simulink model "Model_GBXCluctchOpt_V5"  (R2024b)
settings: Solver=VariableStepAuto  StartTime=0.0  StopTime=552  RelTol=1e-5
undefined symbols (not defined in the file): Bdy_facCoG_C, Bdy_facTireFric_C, Bdy_lenRadiusWheel_C, Bdy_lenWheelBase_C, Bdy_lenZCoG_C, Bdy_mEquivalentJ_C, Bdy_mVeh_C, Bdy_vsqr2frc_C, Drv_kmh2gradtqDriver_C, Drv_kmh2tqDriver_C, Edr_pwr_LossMap_AXIS, Edr_pwrInverterLosses_MAP, Edr_pwrMachineLosses_MAP, Edr_rpm_InvLossMap_AXIS, Edr_rpm_MachLossMap_AXIS, Edr_rpm_MaxMinTq_AXIS, Edr_rpmMax_C, Edr_tq_MachLossMap_AXIS, Edr_tqEffMax_CUR, Env_facSlope_WLTC_CUR, Env_facSlopeBAB185_CUR, Env_facSlopeCrossCountry_CUR, Env_kmhDesBAB185_CUR, Env_kmhDesCrossCountry_CUR, Env_vVehDes_NEDC_kmh, Env_vVehDes_WLTC_kmh, Env_vVehTime_NEDC_s, Env_vVehTime_WLTC_s, Gbx_facGbxRatioRe_C, Ice_derfacLoadDecrease_MAP, Ice_derfacLoadIncrease_MAP, Ice_etaLam_CUR, Ice_facEtaCocMax_MAP, Ice_facFuelEnRich_MAP, Ice_KUMSRL_C, Ice_Lambda_AXIS, Ice_relLoad2relTqOptIgnLamOne_MAP, Ice_relLoad_AXIS, Ice_relLoad_LoadDyn_AXIS, Ice_relLoad_Max_CUR, Ice_relTq_AXIS, Ice_relTqInr2TqInr_C, Ice_relTqOptIgnLamOne2relLoad_MAP, Ice_rpm_AXIS, Ice_rpm_LoadDyn_AXIS, Ice_rpm_relLoadMax_AXIS, Ice_tqLossesIce_MAP, Pnt_capBat_C, Pnt_facSocBatOcv_AXIS, Pnt_facSocInit_C, Pnt_iBatChrgMax_C, Pnt_iBatDisChrgMax_C, Pnt_resBatInner_C, Pnt_uBatMax_C, Pnt_uBatMin_C, Pnt_uBatOcv_CUR, Vco_flgEdrExists_CFG, Vco_flgIceCluAlwClosed_CFG, Vco_flgIceExists_CFG
libraries: simulink x7, simulink_extras x6
(part 2 of 3)

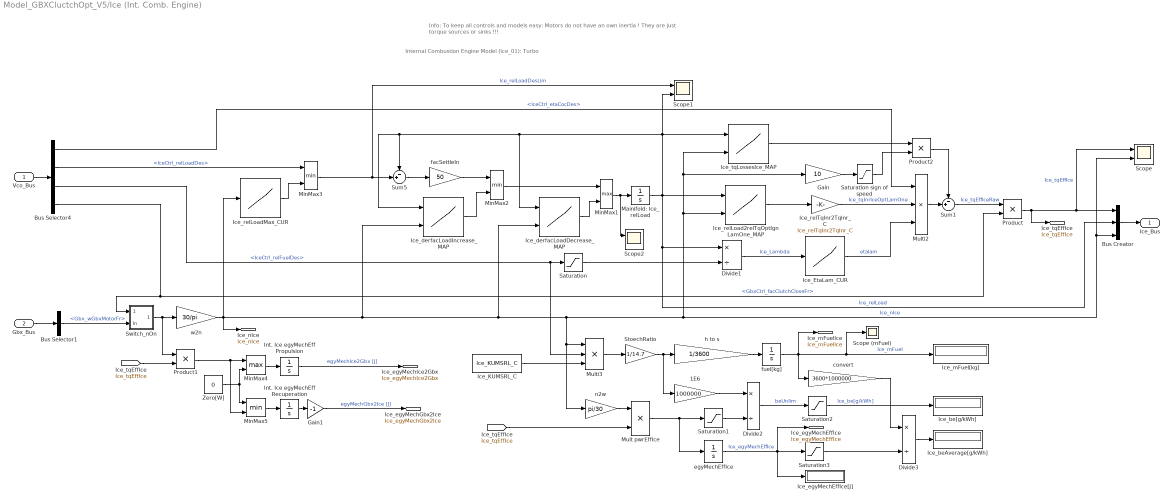
== system Model_GBXCluctchOpt_V5/Ice (Int. Comb. Engine) ==
  note: Internal Combustion Engine Model (Ice_01): Turbo
  note: Info: To keep all controls and models easy: Motors do not have an own inertia !
      | They are just torque sources or sinks !!!
  Vco_Bus : Inport
  Gbx_Bus : Inport  Port=2
  " h to s" : Gain  Gain=1/3600
  1E6 : Gain  Gain=1000000
  Bus Creator : BusCreator  Inputs=3
  Bus Selector1 : BusSelector  OutputSignals=Gbx_wGbxMotorFr
  Bus Selector4 : BusSelector  OutputSignals=IceCtrl_etaCocDes,IceCtrl_relLoadDes,IceCtrl_relFuelDes,GbxCtrl_facClutchCloseFr
  Divide1 : Product  Inputs=*/
  Divide2 : Product  Inputs=*/
  Divide3 : Product  Inputs=*/
  Gain : Gain  Gain=10
  Gain1 : Gain  Gain=-1
  Ice_EtaLam_CUR : Lookup_n-D  NumberOfTableDimensions=1  BreakpointsForDimension1=Ice_Lambda_AXIS  Table=Ice_etaLam_CUR  ExtrapMethod=Clip  InternalRulePriority=Speed  RndMeth=Simplest
  Ice_KUMSRL_C : Constant  Value=Ice_KUMSRL_C
  Ice_beAverage[g/kWh] : Display
  Ice_be[g/kWh] : Display
  Ice_derfacLoadDecrease_MAP : Lookup_n-D  BreakpointsForDimension1=Ice_relLoad_LoadDyn_AXIS  BreakpointsForDimension2=Ice_rpm_LoadDyn_AXIS  Table=Ice_derfacLoadDecrease_MAP  ExtrapMethod=Clip  UseLastTableValue=on  InternalRulePriority=Speed  RndMeth=Simplest
      settings: InputPortMap=u0,u1
  Ice_derfacLoadIncrease_MAP : Lookup_n-D  BreakpointsForDimension1=Ice_relLoad_LoadDyn_AXIS  BreakpointsForDimension2=Ice_rpm_LoadDyn_AXIS  Table=Ice_derfacLoadIncrease_MAP  ExtrapMethod=Clip  UseLastTableValue=on  InternalRulePriority=Speed  RndMeth=Simplest
      settings: InputPortMap=u0,u1
  Ice_egyMechEffIce[J] : Display
  Ice_mFuel[kg] : Display
  Ice_relLoad2relTqOptIgnLamOne_MAP : Lookup_n-D  BreakpointsForDimension1=Ice_relLoad_AXIS  BreakpointsForDimension2=Ice_rpm_AXIS  Table=Ice_relLoad2relTqOptIgnLamOne_MAP  ExtrapMethod=Clip  InternalRulePriority=Speed  RndMeth=Simplest
      settings: InputPortMap=u0,u1
  Ice_relLoadMax_CUR : Lookup_n-D  NumberOfTableDimensions=1  BreakpointsForDimension1=Ice_rpm_relLoadMax_AXIS  Table=Ice_relLoad_Max_CUR  ExtrapMethod=Clip  InternalRulePriority=Speed  RndMeth=Simplest
  Ice_relTqInr2TqInr_C : Gain  Gain=Ice_relTqInr2TqInr_C
  Ice_tqLossesIce_MAP : Lookup_n-D  BreakpointsForDimension1=Ice_relLoad_AXIS  BreakpointsForDimension2=Ice_rpm_AXIS  Table=Ice_tqLossesIce_MAP  ExtrapMethod=Clip  InternalRulePriority=Speed  RndMeth=Simplest
      settings: InputPortMap=u0,u1
  Int. Ice egyMechEff Propulsion : Integrator
  Int. Ice egyMechEff Recuperation : Integrator
  Mainifold: Ice_relLoad : Integrator  InitialCondition=80  LimitOutput=on  LowerSaturationLimit=0
  MinMax1 : MinMax  Function=max  Inputs=2
  MinMax2 : MinMax  Inputs=2
  MinMax3 : MinMax  Inputs=2
  MinMax4 : MinMax  Function=max  Inputs=2  ZeroCross=off
  MinMax5 : MinMax  Inputs=2  ZeroCross=off
  Mult pwrEffIce : Product  Inputs=**
  Multi2 : Product  Inputs=***
  Multi3 : Product  Inputs=***
  Product : Product
  Product1 : Product
  Product2 : Product
  Saturation : Saturate  UpperLimit=1000  LowerLimit=0.0001
  Saturation sign of speed : Saturate  UpperLimit=1  LowerLimit=-1
  Saturation1 : Saturate  UpperLimit=inf  LowerLimit=0.1
  Saturation2 : Saturate  UpperLimit=1000  LowerLimit=0
  Saturation3 : Saturate  UpperLimit=inf  LowerLimit=0.1
  Scope : Scope  NumInputPorts=2
  "Scope (mFuel) " : Scope
  Scope1 : Scope  NumInputPorts=2
  Scope2 : Scope  NumInputPorts=2
  StoechRatio : Gain  Gain=1/14.7
  Sum1 : Sum  Inputs=-+|
  Sum5 : Sum  Inputs=-+|
  Switch_nOn : Subsystem
  "Zero[W] " : Constant  Value=0
  convert : Gain  Gain=3600*1000000
  egyMechEffIce : Integrator
  facSettleIn : Gain  Gain=50
  fuel[kg] : Integrator
  n2w : Gain  Gain=pi/30
  "w2n  " : Gain  Gain=30/pi
  Ice_Bus : Outport  VectorParamsAs1DForOutWhenUnconnected=off
  tag scope: Ice_egyMechEffIce=global, Ice_egyMechGbx2Ice=global, Ice_egyMechIce2Gbx=global, Ice_mFuelIce=global, Ice_nIce=global, Ice_tqEffIce=global
  wires:
  Bus Creator/1 -> Ice_Bus/1
  Vco_Bus/1 -> Bus Selector4/1
  Product/1 -> [Ice_tqEffIce], Bus Creator/1, Scope/1  "Ice_tqEffIce"
  Gbx_Bus/1 -> Bus Selector1/1
  "w2n  "/1 -> [Ice_nIce], Ice_relLoadMax_CUR/1, Ice_derfacLoadDecrease_MAP/2, n2w/1, Multi3/1, Gain/1, Ice_tqLossesIce_MAP/2, Ice_relLoad2relTqOptIgnLamOne_MAP/2, Scope/2, Bus Creator/3, Ice_derfacLoadIncrease_MAP/2  "Ice_nIce"
  Bus Selector1/1 -> Switch_nOn/2(In)  "<Gbx_wGbxMotorFr>"
  Mainifold: Ice_relLoad/1 -> Bus Creator/2, Divide1/1, Ice_relLoad2relTqOptIgnLamOne_MAP/1, Scope1/2, Ice_tqLossesIce_MAP/1, Ice_derfacLoadDecrease_MAP/1, Ice_derfacLoadIncrease_MAP/1, Sum5/1  "Ice_relLoad"
  Ice_relLoadMax_CUR/1 -> MinMax3/2
  Bus Selector4/2 -> MinMax3/1  "<IceCtrl_relLoadDes>"
  Bus Selector4/1 -> Multi2/1  "<IceCtrl_etaCocDes>"
  Bus Selector4/3 -> Multi3/2, Saturation/1  "<IceCtrl_relFuelDes>"
  Ice_derfacLoadIncrease_MAP/1 -> MinMax2/2
  Ice_derfacLoadDecrease_MAP/1 -> MinMax1/2
  MinMax2/1 -> MinMax1/1
  MinMax1/1 -> Scope2/1, Mainifold: Ice_relLoad/1
  Sum5/1 -> facSettleIn/1
  facSettleIn/1 -> MinMax2/1
  MinMax3/1 -> Scope1/1, Sum5/2  "Ice_relLoadDesLim"
  Saturation/1 -> Divide1/2
  Divide1/1 -> Ice_EtaLam_CUR/1  "Ice_Lambda"
  Ice_relLoad2relTqOptIgnLamOne_MAP/1 -> Ice_relTqInr2TqInr_C/1
  Ice_relTqInr2TqInr_C/1 -> Multi2/2  "Ice_tqInrIceOptLamOne"
  Ice_EtaLam_CUR/1 -> Multi2/3  "etalam"
  Multi2/1 -> Sum1/2
  Ice_tqLossesIce_MAP/1 -> Product2/1
  Sum1/1 -> Product/1  "Ice_tqEffIceRaw"
  Bus Selector4/4 -> Switch_nOn/1(flag), Product/2  "<GbxCtrl_facClutchCloseFr>"
  Int. Ice egyMechEff Recuperation/1 -> Gain1/1
  MinMax5/1 -> Int. Ice egyMechEff Recuperation/1
  "Zero[W] "/1 -> MinMax5/1, MinMax4/2
  Product1/1 -> MinMax4/1, MinMax5/2
  MinMax4/1 -> Int. Ice egyMechEff Propulsion/1
  Gain1/1 -> [Ice_egyMechGbx2Ice]  "egyMechGbx2Ice [J]"
  Int. Ice egyMechEff Propulsion/1 -> [Ice_egyMechIce2Gbx]  "egyMechIce2Gbx [J]"
  [Ice_tqEffIce] -> Product1/2
  Switch_nOn/1(Out) -> Product1/1, "w2n  "/1
  Product2/1 -> Sum1/1
  Saturation sign of speed/1 -> Product2/2
  Gain/1 -> Saturation sign of speed/1
  Ice_KUMSRL_C/1 -> Multi3/3
  Multi3/1 -> StoechRatio/1
  StoechRatio/1 -> 1E6/1, " h to s"/1
  " h to s"/1 -> fuel[kg]/1
  fuel[kg]/1 -> convert/1, [Ice_mFuelIce], "Scope (mFuel) "/1, Ice_mFuel[kg]/1  "Ice_mFuel"
  [Ice_tqEffIce] -> Mult pwrEffIce/2
  n2w/1 -> Mult pwrEffIce/1
  Mult pwrEffIce/1 -> egyMechEffIce/1, Saturation1/1
  Saturation1/1 -> Divide2/2
  1E6/1 -> Divide2/1
  Divide2/1 -> Saturation2/1  "beUnlim"
  Saturation2/1 -> Ice_be[g/kWh]/1  "Ice_be[g/kWh]"
  egyMechEffIce/1 -> [Ice_egyMechEffIce], Ice_egyMechEffIce[J]/1, Saturation3/1  "Ice_egyMechEffIce"
  Saturation3/1 -> Divide3/2
  convert/1 -> Divide3/1
  Divide3/1 -> Ice_beAverage[g/kWh]/1

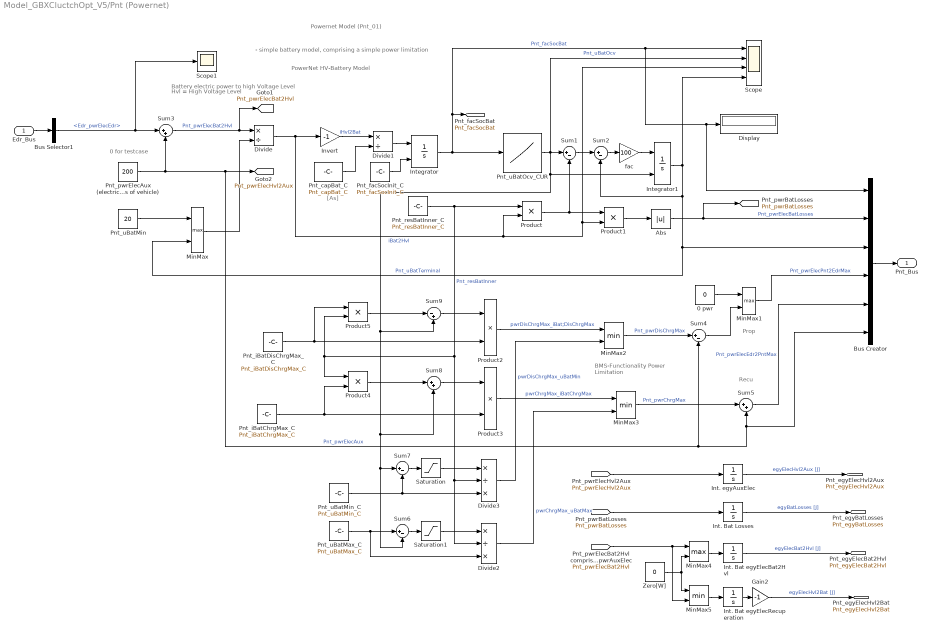
== system Model_GBXCluctchOpt_V5/Pnt (Powernet) ==
  note: Prop
  note: 0 for testcase
  note: [As]
  note: Powernet Model (Pnt_01)
  note: PowerNet HV-Battery Model
  note: Battery electric power to high Voltage Level
  note: Recu
  note: - simple battery model, comprising a simple power limitation
  note: BMS-Functionality
      | Power Limitation
  note: Hvl = High Voltage Level
  Edr_Bus : Inport
  0 pwr : Constant  Value=0
  Abs : Abs  SaturateOnIntegerOverflow=off
  Bus Creator : BusCreator  Inputs=6
  Bus Selector1 : BusSelector  OutputSignals=Edr_pwrElecEdr
  Display : Display
  Divide : Product  Inputs=*/
  Divide1 : Product  Inputs=*/
  Divide2 : Product  Inputs=*/*
  Divide3 : Product  Inputs=*/*
  Gain2 : Gain  Gain=-1
  Int. Bat Losses : Integrator
  Int. Bat egyElecBat2Hvl : Integrator
  Int. Bat egyElecRecuperation : Integrator
  Int. egyAuxElec : Integrator
  Integrator : Integrator  InitialConditionSource=external  InitialCondition=0.8  LimitOutput=on  UpperSaturationLimit=1  LowerSaturationLimit=0
  Integrator1 : Integrator  InitialConditionSource=external  InitialCondition=0.8
  Invert : Gain  Gain=-1
  MinMax : MinMax  Function=max  Inputs=2
  MinMax1 : MinMax  Function=max  Inputs=2
  MinMax2 : MinMax  Inputs=2
  MinMax3 : MinMax  Inputs=2
  MinMax4 : MinMax  Function=max  Inputs=2  ZeroCross=off
  MinMax5 : MinMax  Inputs=2  ZeroCross=off
  Pnt_capBat_C : Constant  Value=Pnt_capBat_C
  Pnt_facSocInit_C : Constant  Value=Pnt_facSocInit_C
  Pnt_iBatChrgMax_C : Constant  Value=Pnt_iBatChrgMax_C
  Pnt_iBatDisChrgMax_C : Constant  Value=Pnt_iBatDisChrgMax_C
  Pnt_pwrElecAux (electric auxilliaries of vehicle) : Constant  Value=200
  Pnt_resBatInner_C : Constant  Value=Pnt_resBatInner_C
  Pnt_uBatMax_C : Constant  Value=Pnt_uBatMax_C
  Pnt_uBatMin : Constant  Value=20
  Pnt_uBatMin_C : Constant  Value=Pnt_uBatMin_C
  Pnt_uBatOcv_CUR : Lookup  InputValues=Pnt_facSocBatOcv_AXIS  Table=Pnt_uBatOcv_CUR  LookUpMeth=Interpolation-Use End Values  SaturateOnIntegerOverflow=off
  Product : Product  RndMeth=Zero
  Product1 : Product  RndMeth=Zero
  Product{2..5} (4 alike) : Product
  Saturation : Saturate  UpperLimit=1000  LowerLimit=0
  Saturation1 : Saturate  UpperLimit=1000  LowerLimit=0
  Scope : Scope  NumInputPorts=4
  Scope1 : Scope
  Sum{1..2,4,6..7} (5 alike) : Sum  Inputs=|+-
  Sum3 : Sum  Inputs=|++
  Sum5 : Sum  Inputs=|++
  Sum8 : Sum  Inputs=|++
  Sum9 : Sum  Inputs=|-+
  Zero[W] : Constant  Value=0
  fac : Gain  Gain=100
  Pnt_Bus : Outport  VectorParamsAs1DForOutWhenUnconnected=off
  tag scope: Pnt_egyBatLosses=global, Pnt_egyElecBat2Hvl=global, Pnt_egyElecHvl2Aux=global, Pnt_egyElecHvl2Bat=global, Pnt_facSocBat=global, Pnt_pwrBatLosses=global, Pnt_pwrElecBat2Hvl=global, Pnt_pwrElecHvl2Aux=global
  wires:
  Bus Creator/1 -> Pnt_Bus/1
  Sum5/1 -> Bus Creator/5  "Pnt_pwrElecEdr2PntMax"
  MinMax1/1 -> Bus Creator/4  "Pnt_pwrElecPnt2EdrMax"
  Int. egyAuxElec/1 -> [Pnt_egyElecHvl2Aux]  "egyElecHvl2Aux [J]"
  Int. Bat Losses/1 -> [Pnt_egyBatLosses]  "egyBatLosses [J]"
  [Pnt_pwrElecHvl2Aux] -> Int. egyAuxElec/1
  Pnt_iBatDisChrgMax_C/1 -> Product5/1, Product2/2
  Sum8/1 -> Product3/1
  Zero[W]/1 -> MinMax5/1, MinMax4/2
  [Pnt_pwrBatLosses] -> Int. Bat Losses/1
  0 pwr/1 -> MinMax1/1
  Pnt_iBatChrgMax_C/1 -> Product4/2, Product3/2
  Saturation1/1 -> Divide2/1
  Pnt_pwrElecAux (electric auxilliaries of vehicle)/1 -> Sum5/2, Bus Creator/6, Sum4/2, [Pnt_pwrElecHvl2Aux], Sum3/2  "Pnt_pwrElecAux"
  Divide/1 -> Invert/1, Product/2, Scope/3, Product1/2  "iBat2Hvl"
  Pnt_uBatMax_C/1 -> Divide2/3, Sum6/1
  MinMax5/1 -> Int. Bat egyElecRecuperation/1
  Sum6/1 -> Saturation1/1
  Gain2/1 -> [Pnt_egyElecHvl2Bat]  "egyElecHvl2Bat [J]"
  Sum1/1 -> Sum2/1
  Int. Bat egyElecRecuperation/1 -> Gain2/1
  Int. Bat egyElecBat2Hvl/1 -> [Pnt_egyElecBat2Hvl]  "egyElecBat2Hvl [J]"
  MinMax/1 -> Divide/2
  Sum3/1 -> [Pnt_pwrElecBat2Hvl], Divide/1  "Pnt_pwrElecBat2Hvl"
  Divide3/1 -> MinMax2/2  "pwrDisChrgMax_uBatMin"
  Product5/1 -> Sum9/1
  Divide2/1 -> MinMax3/2  "pwrChrgMax_uBatMax"
  Sum7/1 -> Saturation/1
  Product4/1 -> Sum8/1
  MinMax4/1 -> Int. Bat egyElecBat2Hvl/1
  Sum2/1 -> fac/1
  Integrator1/1 -> MinMax/2, Bus Creator/3, Sum2/2, Scope/4  "Pnt_uBatTerminal"
  MinMax3/1 -> Sum5/1  "Pnt_pwrChrgMax"
  Product3/1 -> MinMax3/1  "pwrChrgMax_iBatChrgMax"
  Abs/1 -> [Pnt_pwrBatLosses], Bus Creator/2  "Pnt_pwrElecBatLosses"
  MinMax2/1 -> Sum4/1  "Pnt_pwrDisChrgMax"
  Pnt_uBatOcv_CUR/1 -> Scope/2, Sum9/2, Sum8/2, Sum6/2, Sum7/1, Integrator1/2, Sum1/1  "Pnt_uBatOcv"
  fac/1 -> Integrator1/1
  Product2/1 -> MinMax2/1  "pwrDisChrgMax_iBat;DisChrgMax"
  Pnt_resBatInner_C/1 -> Divide2/2, Divide3/2, Product4/1, Product5/2, Product/1  "Pnt_resBatInner"
  Sum9/1 -> Product2/1
  Product/1 -> Product1/1, Sum1/2
  [Pnt_pwrElecBat2Hvl] -> MinMax4/1, MinMax5/2
  Invert/1 -> Divide1/1  "iHvl2Bat"
  Bus Selector1/1 -> Sum3/1, Scope1/1  "<Edr_pwrElecEdr>"
  Integrator/1 -> Pnt_uBatOcv_CUR/1, Display/1, Bus Creator/1, Scope/1, [Pnt_facSocBat]  "Pnt_facSocBat"
  Sum4/1 -> MinMax1/2
  Product1/1 -> Abs/1
  Pnt_uBatMin_C/1 -> Sum7/2, Divide3/3
  Divide1/1 -> Integrator/1
  Saturation/1 -> Divide3/1
  Pnt_uBatMin/1 -> MinMax/1
  Pnt_facSocInit_C/1 -> Integrator/2
  Pnt_capBat_C/1 -> Divide1/2
  Edr_Bus/1 -> Bus Selector1/1

== system Model_GBXCluctchOpt_V5/Vco (Vehicle Control) ==
  note: GbxCtrl shall comprise the calculation of the desired torques for the motors, it shall respect the max. torque that can be transferred to the road.
  note: Vehicle Control Model (Vco_Hybrid_01)
      | Variant - for P4 Hybrid with
      | - Rear Axel Central Drive, Fixed Gear Ratio for E-Machine
      | - Front Axle Central Drive,  5 Gear Transmission
  note: E-Drive Control (EdrCtrl)
  note: Brake-Drive Control (BrkCtrl)
  note: Int. Comb. Eng. Control (IceCtrl)
  note: Main Control + Gearbox Control
  note: Ice => Gbx Front
      | Edr => Gbx Rear
  Ice_Bus : Inport
  Edr_Bus : Inport  Port=2
  Pnt_Bus : Inport  Port=3
  Drv_Bus : Inport  Port=4
  Bdy_Bus : Inport  Port=5
  Gbx_Bus : Inport  Port=6
  BrkCtrl : Subsystem
  Bus Creator : BusCreator  Inputs=9
  Bus Selector1 : BusSelector  OutputSignals=Drv_kmhVehDesLim,Drv_tqDrvWheelAxDes
  Bus Selector2 : BusSelector  OutputSignals=Pnt_facSocBat,Pnt_pwrElecEdr2PntMax,Pnt_pwrElecPnt2EdrMax
  Bus Selector3 : BusSelector  OutputSignals=Bdy_tqAbsMaxAxFr,Bdy_tqAbsMaxAxRe,Bdy_kmhVeh
  Bus Selector4 : BusSelector  OutputSignals=Gbx_facGbxRatioFr,Gbx_facGbxRatioRe,Gbx_tqGbxAxFr,Gbx_tqGbxAxRe
  Bus Selector5 : BusSelector  OutputSignals=Ice_relLoad,Ice_nIce,Ice_tqEffIce
  Bus Selector6 : BusSelector  OutputSignals=Edr_nEdr
  EdrCtrl : Subsystem
  IceCtrl : Subsystem
  MainCtrl (Comb) : Subsystem  Commented=on
  MainCtrl (Hybrid) : Subsystem
  MainCtrl (Pure EV) : Subsystem  Commented=on
  Vco_Bus : Outport  VectorParamsAs1DForOutWhenUnconnected=off
  wires:
  Bus Creator/1 -> Vco_Bus/1
  Drv_Bus/1 -> Bus Selector1/1
  Pnt_Bus/1 -> Bus Selector2/1
  Gbx_Bus/1 -> Bus Selector4/1
  Ice_Bus/1 -> Bus Selector5/1
  Bus Selector2/2 -> EdrCtrl/3(<Pnt_pwrElecEdr2PntMax>)  "<Pnt_pwrElecEdr2PntMax>"
  Bus Selector2/3 -> EdrCtrl/4(<Pnt_pwrElecPnt2EdrMax>)  "<Pnt_pwrElecPnt2EdrMax>"
  EdrCtrl/1(EdrCtrl_tqEdrLimDes) -> Bus Creator/7  "EdrCtrl_tqEdrLimDes"
  IceCtrl/1(IceCtrl_tqEffIceLimDes) -> Bus Creator/1  "IceCtrl_tqEffIceLimDes"
  Bus Selector1/2 -> BrkCtrl/3(Drv_tqWheelAxDes), MainCtrl (Hybrid)/3(<Drv_tqDrvWheelAxlDes>)  "<Drv_tqDrvWheelAxDes>"
  MainCtrl (Hybrid)/1(MainCtrl_tqEffIceDes) -> IceCtrl/3(MainCtrl_tqEffIceDes)
  MainCtrl (Hybrid)/5(MainCtrl_tqEdrDes) -> EdrCtrl/1(MainCtrl_tqEdrDes)
  Bus Selector4/1 -> MainCtrl (Hybrid)/4(<Gbx_facGbxRatioFr>)  "<Gbx_facGbxRatioFr>"
  Bus Selector4/2 -> MainCtrl (Hybrid)/5(<Gbx_facGbxRatioRe>)  "<Gbx_facGbxRatioRe>"
  MainCtrl (Hybrid)/3(GbxCtrl_numGearAxFrDes) -> Bus Creator/5  "GbxCtrl_numGearAxFrDes"
  MainCtrl (Hybrid)/4(GbxCtrl_facClutchCloseFr) -> Bus Creator/6  "GbxCtrl_facClutchCloseFr"
  BrkCtrl/2(Vco_tqBrkAxlReDes) -> Bus Creator/9  "BrkCtrl_tqBrkAxReDes"
  BrkCtrl/1(Vco_tqBrkAxlFrDes) -> Bus Creator/8  "BrkCtrl_tqBrkAxFrDes"
  Bus Selector4/3 -> BrkCtrl/6(Gbx_tqAxFr)  "<Gbx_tqGbxAxFr>"
  Bus Selector4/4 -> BrkCtrl/7(Gbx_tqAxRe)  "<Gbx_tqGbxAxRe>"
  Bdy_Bus/1 -> Bus Selector3/1
  Bus Selector3/1 -> MainCtrl (Hybrid)/6(<Bdy_tqAbsMaxAxFr>), BrkCtrl/5(Bdy_tqAbsMaxAxFr)  "<Bdy_tqAbsMaxAxFr>"
  Bus Selector3/2 -> MainCtrl (Hybrid)/7(<Bdy_tqAbsMaxAxRe>), BrkCtrl/4(Bdy_tqAbsMaxAxRe)  "<Bdy_tqAbsMaxAxRe>"
  IceCtrl/6(IceCtrl_tqEffIceMin) -> MainCtrl (Hybrid)/12(<IceCtrl_tqEffIceMin>)
  IceCtrl/5(IceCtrl_tqEffIceMax) -> MainCtrl (Hybrid)/11(<IceCtrl_tqEffIceMax>)
  EdrCtrl/3(EdrCtrl_tqEdrMin) -> MainCtrl (Hybrid)/10(<EdrCtrl_tqEdrMin>)
  EdrCtrl/2(EdrCtrl_tqEdrMax) -> MainCtrl (Hybrid)/9(<EdrCtrl_tqEdrMax>)
  Edr_Bus/1 -> Bus Selector6/1
  Bus Selector1/1 -> BrkCtrl/2(Drv_kmhVehDesLim), MainCtrl (Hybrid)/2(<Drv_kmhVehDesLim>)  "<Drv_kmhVehDesLim>"
  Bus Selector3/3 -> MainCtrl (Hybrid)/8(Bdy_kmhVeh), BrkCtrl/1(Bdy_kmhVeh)  "<Bdy_kmhVeh>"
  MainCtrl (Hybrid)/2(MainCtrl_flgIceOn) -> IceCtrl/4(MainCtrl_flgIceOn)
  Bus Selector5/2 -> IceCtrl/2(Ice_nIce)  "<Ice_nIce>"
  Bus Selector5/1 -> IceCtrl/1(Ice_relLoad)  "<Ice_relLoad>"
  IceCtrl/2(IceCtrl_relLoadDes) -> Bus Creator/2  "IceCtrl_relLoadDes"
  IceCtrl/3(IceCtrl_etaCocDes) -> Bus Creator/3  "IceCtrl_etaCocDes"
  IceCtrl/4(IceCtrl_relFuelDes) -> Bus Creator/4  "IceCtrl_relFuelDes"
  Bus Selector5/3 -> MainCtrl (Hybrid)/1(Ice_tqEffIce)  "<Ice_tqEffIce>"
  Bus Selector6/1 -> EdrCtrl/2(Edr_nEdr)  "<Edr_nEdr>"
  Bus Selector2/1 -> MainCtrl (Hybrid)/13(Pnt_facSocBat)  "<Pnt_facSocBat>"

== system Model_GBXCluctchOpt_V5/Env (Environment)/Filter ==
  in : Inport
  Scope1 : Scope  NumInputPorts=3
  Transfer Fcn : TransferFcn  Denominator=[0.1 1]
  Transfer Fcn1 : TransferFcn  Denominator=[0.1 1]
  out : Outport
  wires:
  in/1 -> Scope1/1, Transfer Fcn/1
  Transfer Fcn/1 -> Scope1/2, Transfer Fcn1/1
  Transfer Fcn1/1 -> out/1, Scope1/3  "Env_kmhVehDes [km/h]"

== system Model_GBXCluctchOpt_V5/Gbx (Gear Box)/Ramp ==
  in : Inport
  Gain : Gain  Gain=10000
  Integrator : Integrator  InitialCondition=1
  Saturation : Saturate  UpperLimit=10  LowerLimit=-10
  Sum2 : Sum  Inputs=|+-
  Out : Outport
  wires:
  Integrator/1 -> Sum2/2, Out/1
  in/1 -> Sum2/1
  Sum2/1 -> Gain/1
  Saturation/1 -> Integrator/1
  Gain/1 -> Saturation/1

== system Model_GBXCluctchOpt_V5/Gbx (Gear Box)/tqLoss GbxFrontExists ==
  w : Inport
  tqIn : Inport  Port=2
  Gain : Gain  Gain=1000
  Product7 : Product  Inputs=3
  Saturation sign of speed : Saturate  UpperLimit=1  LowerLimit=-1
  Vco_flgIceExists_CFG : Constant  Value=Vco_flgIceExists_CFG
  tqOut : Outport
  wires:
  Gain/1 -> Saturation sign of speed/1
  w/1 -> Gain/1
  Product7/1 -> tqOut/1
  Saturation sign of speed/1 -> Product7/1
  tqIn/1 -> Product7/2
  Vco_flgIceExists_CFG/1 -> Product7/3

== system Model_GBXCluctchOpt_V5/Gbx (Gear Box)/tqLoss GbxRearExists ==
  tqIn : Inport
  w : Inport  Port=2
  Gain : Gain  Gain=1000
  Product7 : Product  Inputs=3
  Saturation sign of speed : Saturate  UpperLimit=1  LowerLimit=-1
  Vco_flgEdrExists_CFG : Constant  Value=Vco_flgEdrExists_CFG
  tqOut : Outport
  wires:
  Gain/1 -> Saturation sign of speed/1
  w/1 -> Gain/1
  Product7/1 -> tqOut/1
  Saturation sign of speed/1 -> Product7/1
  tqIn/1 -> Product7/2
  Vco_flgEdrExists_CFG/1 -> Product7/3

== system Model_GBXCluctchOpt_V5/Ice (Int. Comb. Engine)/Switch_nOn ==
  flag : Inport
  In : Inport  Port=2
  Constant : Constant  Value=0
  Switch : Switch  Criteria=u2 > Threshold  Threshold=0.5  SaturateOnIntegerOverflow=off  InputSameDT=off
  Out : Outport
  wires:
  Switch/1 -> Out/1
  flag/1 -> Switch/2
  Constant/1 -> Switch/3
  In/1 -> Switch/1

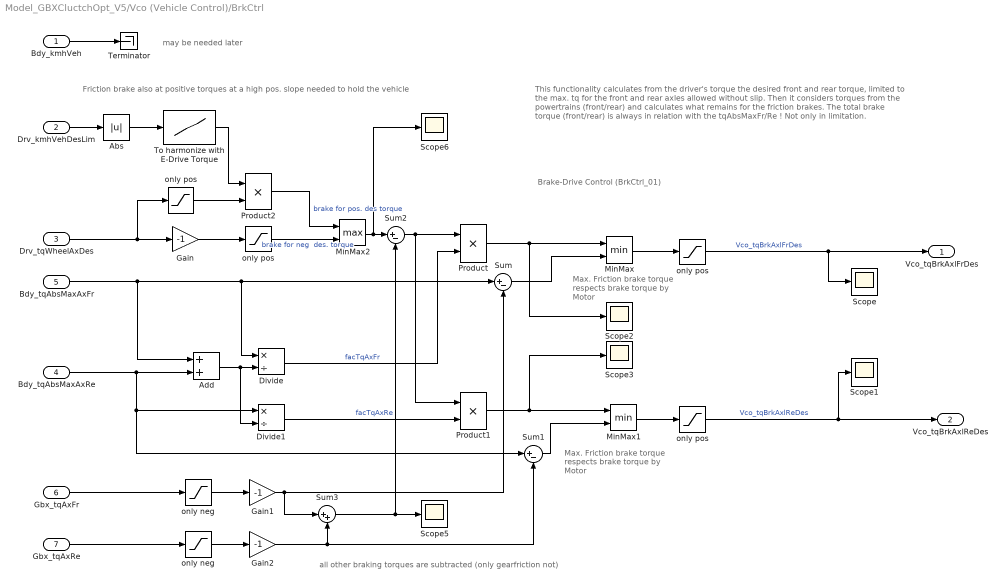
== system Model_GBXCluctchOpt_V5/Vco (Vehicle Control)/BrkCtrl ==
  note: all other braking torques are subtracted (only gearfriction not)
  note: Friction brake also at positive torques at a high pos. slope needed to hold the vehicle
  note: Max. Friction brake torque
      | respects brake torque by Motor
  note: This functionality calculates from the driver's torque the desired front and rear torque, limited to the max. tq for the front and rear axles allowed without slip.
      |
      | Then it considers torques from the powertrains (front/rear) and calculates what remains for the friction brakes.
      |
      | The total brake torque (front/rear) is always in relation with the tqAbsMaxFr/Re !
      | Not only in limitation.
  note: Max. Friction brake torque
      | respects brake torque by Motor
  note: Brake-Drive Control (BrkCtrl_01)
  note: may be needed later
  Bdy_kmhVeh : Inport
  Drv_kmhVehDesLim : Inport  Port=2
  Drv_tqWheelAxDes : Inport  Port=3
  Bdy_tqAbsMaxAxRe : Inport  Port=4
  Bdy_tqAbsMaxAxFr : Inport  Port=5
  Gbx_tqAxFr : Inport  Port=6
  Gbx_tqAxRe : Inport  Port=7
  "  only pos  " : Saturate  UpperLimit=inf  LowerLimit=0  ZeroCross=off
  Abs : Abs  ZeroCross=off  SaturateOnIntegerOverflow=off
  Add : Sum
  Divide : Product  Inputs=*/
  Divide1 : Product  Inputs=*/
  Gain : Gain  Gain=-1
  Gain1 : Gain  Gain=-1
  Gain2 : Gain  Gain=-1
  MinMax : MinMax  Inputs=2  ZeroCross=off
  MinMax1 : MinMax  Inputs=2  ZeroCross=off
  MinMax2 : MinMax  Function=max  Inputs=2  ZeroCross=off
  Product : Product
  Product1 : Product
  Product2 : Product
  Scope{,1..3,5..6} (6 alike) : Scope
  Sum : Sum  Inputs=|+-
  Sum1 : Sum  Inputs=|+-
  Sum2 : Sum  Inputs=|+-
  Sum3 : Sum  Inputs=|++
  Terminator : Terminator
  To harmonize with E-Drive Torque : Lookup_n-D  NumberOfTableDimensions=1  BreakpointsForDimension1=[-0.1 0 0.05 0.1]  Table="[ 1  1  0  0]"  InternalRulePriority=Speed  RndMeth=Simplest
  only neg : Saturate  UpperLimit=0  LowerLimit=-inf  ZeroCross=off
  "only neg " : Saturate  UpperLimit=0  LowerLimit=-inf  ZeroCross=off
  only pos : Saturate  UpperLimit=inf  LowerLimit=0  ZeroCross=off
  "only pos " : Saturate  UpperLimit=inf  LowerLimit=0  ZeroCross=off
  "only pos  " : Saturate  UpperLimit=inf  LowerLimit=0  ZeroCross=off
  Vco_tqBrkAxlFrDes : Outport
  Vco_tqBrkAxlReDes : Outport  Port=2
  wires:
  Gbx_tqAxFr/1 -> only neg/1
  Gbx_tqAxRe/1 -> "only neg "/1
  Drv_tqWheelAxDes/1 -> Gain/1, "  only pos  "/1
  only neg/1 -> Gain1/1
  "only neg "/1 -> Gain2/1
  Bdy_tqAbsMaxAxFr/1 -> Sum/1, Divide/1, Add/1
  Gain1/1 -> Sum/2, Sum3/1
  Bdy_tqAbsMaxAxRe/1 -> Add/2, Divide1/1, Sum1/1
  Add/1 -> Divide1/2, Divide/2
  Sum2/1 -> Product/1, Product1/1
  Divide/1 -> Product/2  "facTqAxFr"
  Divide1/1 -> Product1/2  "facTqAxRe"
  Gain2/1 -> Sum3/2, Sum1/2
  MinMax1/1 -> "only pos "/1
  Product/1 -> Scope2/1, MinMax/1
  Sum/1 -> MinMax/2
  MinMax/1 -> only pos/1
  Sum1/1 -> MinMax1/2
  Product1/1 -> Scope3/1, MinMax1/1
  Sum3/1 -> Scope5/1, Sum2/2
  "only pos "/1 -> Scope1/1, Vco_tqBrkAxlReDes/1  "Vco_tqBrkAxlReDes"
  only pos/1 -> Scope/1, Vco_tqBrkAxlFrDes/1  "Vco_tqBrkAxlFrDes"
  Drv_kmhVehDesLim/1 -> Abs/1
  "only pos  "/1 -> MinMax2/2  "brake for neg  des. torque"
  Gain/1 -> "only pos  "/1
  MinMax2/1 -> Scope6/1, Sum2/1
  Product2/1 -> MinMax2/1  "brake for pos. des torque"
  "  only pos  "/1 -> Product2/2
  Abs/1 -> To harmonize with E-Drive Torque/1
  To harmonize with E-Drive Torque/1 -> Product2/1
  Bdy_kmhVeh/1 -> Terminator/1

== system Model_GBXCluctchOpt_V5/Vco (Vehicle Control)/EdrCtrl ==
  note: E-Drive Control (EdrCtrl_01)
  MainCtrl_tqEdrDes : Inport
  Edr_nEdr : Inport  Port=2
  <Pnt_pwrElecEdr2PntMax> : Inport  Port=3
  <Pnt_pwrElecPnt2EdrMax> : Inport  Port=4
  Break Loop : TransferFcn  Denominator=[0.01 1]
  Divide : Product  Inputs=*/
  Divide1 : Product  Inputs=*/
  Edr_pwrInverterLosses_MAP : Lookup_n-D  BreakpointsForDimension1=Edr_pwr_LossMap_AXIS  BreakpointsForDimension2=Edr_rpm_InvLossMap_AXIS  Table=Edr_pwrInverterLosses_MAP  ExtrapMethod=Clip  UseLastTableValue=on  InternalRulePriority=Speed  RndMeth=Simplest
      settings: InputPortMap=u0,u1
  Edr_pwrMachineLosses_MAP : Lookup_n-D  BreakpointsForDimension1=Edr_tq_MachLossMap_AXIS  BreakpointsForDimension2=Edr_rpm_MachLossMap_AXIS  Table=Edr_pwrMachineLosses_MAP  ExtrapMethod=Clip  UseLastTableValue=on  InternalRulePriority=Speed  RndMeth=Simplest
      settings: InputPortMap=u0,u1
  Edr_tqEffEdrMax_CUR : Lookup_n-D  NumberOfTableDimensions=1  BreakpointsForDimension1=Edr_rpm_MaxMinTq_AXIS  Table=Edr_tqEffMax_CUR  ExtrapMethod=Clip  InternalRulePriority=Speed  RndMeth=Simplest
  Edr_tqEffEdrMin_CUR : Lookup_n-D  NumberOfTableDimensions=1  BreakpointsForDimension1=Edr_rpm_MaxMinTq_AXIS  Table=-Edr_tqEffMax_CUR  ExtrapMethod=Clip  InternalRulePriority=Speed  RndMeth=Simplest
  Max : MinMax  Function=max  Inputs=3
  Min : MinMax  Inputs=3
  Min1 : MinMax  Inputs=2
  Min2 : MinMax  Function=max  Inputs=2
  Product : Product
  Saturation : Saturate  UpperLimit=inf  LowerLimit=50
  Scope Edr : Scope  NumInputPorts=2
  Scope1 : Scope  NumInputPorts=2
  Sum : Sum  Inputs=|++
  Sum1 : Sum  Inputs=|+-
  Sum2 : Sum  Inputs=|++
  Sum3 : Sum  Inputs=|--
  n2w : Gain  Gain=pi/30
  tqEffMinMaxPnt : Scope  NumInputPorts=2
  EdrCtrl_tqEdrLimDes : Outport
  EdrCtrl_tqEdrMax : Outport  Port=2
  EdrCtrl_tqEdrMin : Outport  Port=3
  wires:
  Divide1/1 -> Min2/2, tqEffMinMaxPnt/2, Max/3
  Edr_nEdr/1 -> Edr_pwrMachineLosses_MAP/2, Edr_pwrInverterLosses_MAP/2, n2w/1, Edr_tqEffEdrMin_CUR/1, Edr_tqEffEdrMax_CUR/1, Scope Edr/1
  Sum2/1 -> Sum3/2, Sum1/2  "Edr_pwrTotalLosses"
  Edr_pwrMachineLosses_MAP/1 -> Sum2/1, Scope1/1, Sum/2
  Product/1 -> Sum/1  "Edr_pwrMechEffEdr"
  Divide/1 -> Min1/2, tqEffMinMaxPnt/1, Min/3
  Saturation/1 -> Divide/2, Divide1/2
  Break Loop/1 -> Edr_pwrMachineLosses_MAP/1, Product/2
  Sum3/1 -> Divide1/1
  Edr_tqEffEdrMax_CUR/1 -> Min1/1, Min/2  "Edr_tqEffEdrMax"
  n2w/1 -> Saturation/1, Product/1  "Edr_wEdr"
  Sum/1 -> Edr_pwrInverterLosses_MAP/1  "Edr_pwrElecEma"
  Edr_pwrInverterLosses_MAP/1 -> Sum2/2, Scope1/2
  Sum1/1 -> Divide/1
  Edr_tqEffEdrMin_CUR/1 -> Max/2, Min2/1  "Edr_tqEffEdrMin"
  Min/1 -> Max/1
  MainCtrl_tqEdrDes/1 -> Min/1
  Max/1 -> Scope Edr/2, EdrCtrl_tqEdrLimDes/1, Break Loop/1  "EdrCtrl_tqEdrDes"
  <Pnt_pwrElecEdr2PntMax>/1 -> Sum3/1
  <Pnt_pwrElecPnt2EdrMax>/1 -> Sum1/1
  Min1/1 -> EdrCtrl_tqEdrMax/1
  Min2/1 -> EdrCtrl_tqEdrMin/1

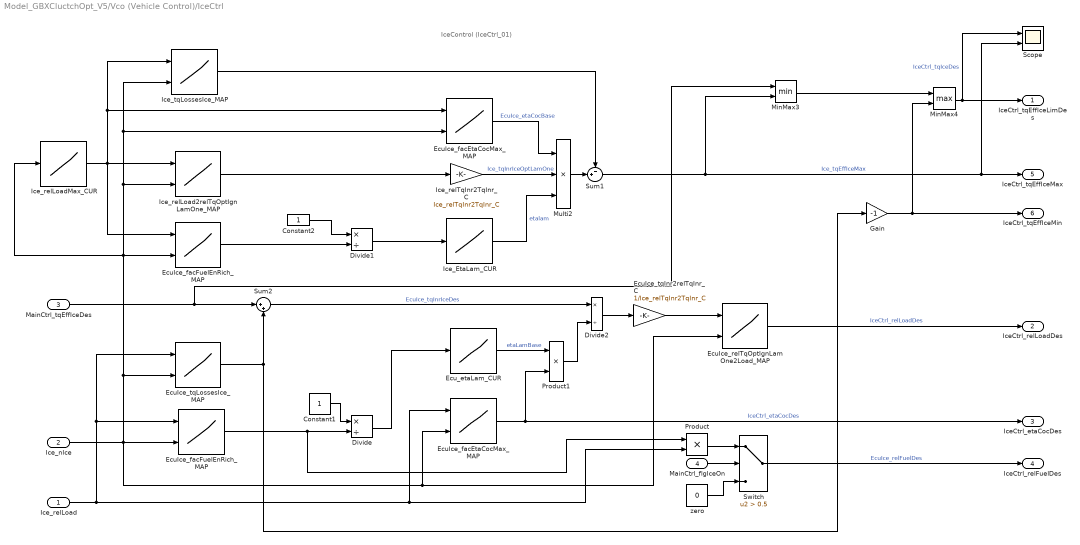
== system Model_GBXCluctchOpt_V5/Vco (Vehicle Control)/IceCtrl ==
  note: IceControl (IceCtrl_01)
  Ice_relLoad : Inport
  Ice_nIce : Inport  Port=2
  MainCtrl_tqEffIceDes : Inport  Port=3
  MainCtrl_flgIceOn : Inport  Port=4
  " zero " : Constant  Value=0
  Constant1 : Constant
  Constant2 : Constant
  Divide : Product  Inputs=*/
  Divide1 : Product  Inputs=*/
  Divide2 : Product  Inputs=*/
  EcuIce_facEtaCocMax_MAP : Lookup_n-D  BreakpointsForDimension1=Ice_relLoad_AXIS  BreakpointsForDimension2=Ice_rpm_AXIS  Table=Ice_facEtaCocMax_MAP  ExtrapMethod=Clip  InternalRulePriority=Speed  RndMeth=Simplest
      settings: InputPortMap=u0,u1
  "EcuIce_facEtaCocMax_MAP " : Lookup_n-D  BreakpointsForDimension1=Ice_relLoad_AXIS  BreakpointsForDimension2=Ice_rpm_AXIS  Table=Ice_facEtaCocMax_MAP  ExtrapMethod=Clip  InternalRulePriority=Speed  RndMeth=Simplest
      settings: InputPortMap=u0,u1
  EcuIce_facFuelEnRich_MAP : Lookup_n-D  BreakpointsForDimension1=Ice_relLoad_AXIS  BreakpointsForDimension2=Ice_rpm_AXIS  Table=Ice_facFuelEnRich_MAP  ExtrapMethod=Clip  InternalRulePriority=Speed  RndMeth=Simplest
      settings: InputPortMap=u0,u1
  "EcuIce_facFuelEnRich_MAP " : Lookup_n-D  BreakpointsForDimension1=Ice_relLoad_AXIS  BreakpointsForDimension2=Ice_rpm_AXIS  Table=Ice_facFuelEnRich_MAP  ExtrapMethod=Clip  InternalRulePriority=Speed  RndMeth=Simplest
      settings: InputPortMap=u0,u1
  EcuIce_relTqOptIgnLamOne2Load_MAP : Lookup_n-D  BreakpointsForDimension1=Ice_relTq_AXIS  BreakpointsForDimension2=Ice_rpm_AXIS  Table=Ice_relTqOptIgnLamOne2relLoad_MAP  ExtrapMethod=Clip  InternalRulePriority=Speed  RndMeth=Simplest
      settings: InputPortMap=u0,u1
  EcuIce_tqInr2relTqInr_C : Gain  Gain=1/Ice_relTqInr2TqInr_C
  EcuIce_tqLossesIce_MAP : Lookup_n-D  BreakpointsForDimension1=Ice_relLoad_AXIS  BreakpointsForDimension2=Ice_rpm_AXIS  Table=Ice_tqLossesIce_MAP  ExtrapMethod=Clip  InternalRulePriority=Speed  RndMeth=Simplest
      settings: InputPortMap=u0,u1
  Ecu_etaLam_CUR : Lookup_n-D  NumberOfTableDimensions=1  BreakpointsForDimension1=Ice_Lambda_AXIS  Table=Ice_etaLam_CUR  ExtrapMethod=Clip  InternalRulePriority=Speed  RndMeth=Simplest
  Gain : Gain  Gain=-1
  Ice_EtaLam_CUR : Lookup_n-D  NumberOfTableDimensions=1  BreakpointsForDimension1=Ice_Lambda_AXIS  Table=Ice_etaLam_CUR  ExtrapMethod=Clip  InternalRulePriority=Speed  RndMeth=Simplest
  Ice_relLoad2relTqOptIgnLamOne_MAP : Lookup_n-D  BreakpointsForDimension1=Ice_relLoad_AXIS  BreakpointsForDimension2=Ice_rpm_AXIS  Table=Ice_relLoad2relTqOptIgnLamOne_MAP  ExtrapMethod=Clip  InternalRulePriority=Speed  RndMeth=Simplest
      settings: InputPortMap=u0,u1
  Ice_relLoadMax_CUR : Lookup_n-D  NumberOfTableDimensions=1  BreakpointsForDimension1=Ice_rpm_relLoadMax_AXIS  Table=Ice_relLoad_Max_CUR  ExtrapMethod=Clip  InternalRulePriority=Speed  RndMeth=Simplest
  Ice_relTqInr2TqInr_C : Gain  Gain=Ice_relTqInr2TqInr_C
  Ice_tqLossesIce_MAP : Lookup_n-D  BreakpointsForDimension1=Ice_relLoad_AXIS  BreakpointsForDimension2=Ice_rpm_AXIS  Table=Ice_tqLossesIce_MAP  ExtrapMethod=Clip  InternalRulePriority=Speed  RndMeth=Simplest
      settings: InputPortMap=u0,u1
  MinMax3 : MinMax  Inputs=2
  MinMax4 : MinMax  Function=max  Inputs=2
  Multi2 : Product  Inputs=***
  Product : Product
  Product1 : Product
  Scope : Scope  NumInputPorts=2
  Sum1 : Sum  Inputs=-+|
  Sum2 : Sum  Inputs=|++
  Switch : Switch  Criteria=u2 > Threshold  Threshold=0.5  SaturateOnIntegerOverflow=off  InputSameDT=off
  IceCtrl_tqEffIceLimDes : Outport
  IceCtrl_relLoadDes : Outport  Port=2
  IceCtrl_etaCocDes : Outport  Port=3
  IceCtrl_relFuelDes : Outport  Port=4
  IceCtrl_tqEffIceMax : Outport  Port=5
  IceCtrl_tqEffIceMin : Outport  Port=6
  wires:
  MinMax4/1 -> IceCtrl_tqEffIceLimDes/1, Scope/1  "IceCtrl_tqIceDes"
  MinMax3/1 -> MinMax4/1
  MainCtrl_tqEffIceDes/1 -> Sum2/1, MinMax3/1
  Sum2/1 -> Divide2/1  "EcuIce_tqInrIceDes"
  Ecu_etaLam_CUR/1 -> Product1/1  "etaLamBase"
  EcuIce_facEtaCocMax_MAP/1 -> Product1/2, IceCtrl_etaCocDes/1  "IceCtrl_etaCocDes"
  EcuIce_tqInr2relTqInr_C/1 -> EcuIce_relTqOptIgnLamOne2Load_MAP/1
  Product1/1 -> Divide2/2
  Divide2/1 -> EcuIce_tqInr2relTqInr_C/1
  Constant1/1 -> Divide/1
  EcuIce_facFuelEnRich_MAP/1 -> Divide/2, Product/1
  Divide/1 -> Ecu_etaLam_CUR/1
  EcuIce_relTqOptIgnLamOne2Load_MAP/1 -> IceCtrl_relLoadDes/1  "IceCtrl_relLoadDes"
  Switch/1 -> IceCtrl_relFuelDes/1  "EcuIce_relFuelDes"
  Product/1 -> Switch/1
  MainCtrl_flgIceOn/1 -> Switch/2
  " zero "/1 -> Switch/3
  Ice_relLoad/1 -> EcuIce_tqLossesIce_MAP/1, EcuIce_facFuelEnRich_MAP/1, EcuIce_facEtaCocMax_MAP/1, Product/2
  Ice_EtaLam_CUR/1 -> Multi2/3  "etalam"
  Ice_relTqInr2TqInr_C/1 -> Multi2/2  "Ice_tqInrIceOptLamOne"
  Ice_relLoad2relTqOptIgnLamOne_MAP/1 -> Ice_relTqInr2TqInr_C/1
  Ice_tqLossesIce_MAP/1 -> Sum1/1
  Multi2/1 -> Sum1/2
  Ice_relLoadMax_CUR/1 -> "EcuIce_facFuelEnRich_MAP "/1, Ice_tqLossesIce_MAP/1, "EcuIce_facEtaCocMax_MAP "/1, Ice_relLoad2relTqOptIgnLamOne_MAP/1
  "EcuIce_facEtaCocMax_MAP "/1 -> Multi2/1  "EcuIce_etaCocBase"
  "EcuIce_facFuelEnRich_MAP "/1 -> Divide1/2
  Constant2/1 -> Divide1/1
  Divide1/1 -> Ice_EtaLam_CUR/1
  Sum1/1 -> MinMax3/2, IceCtrl_tqEffIceMax/1, Scope/2  "Ice_tqEffIceMax"
  Gain/1 -> MinMax4/2, IceCtrl_tqEffIceMin/1
  EcuIce_tqLossesIce_MAP/1 -> Gain/1, Sum2/2
  Ice_nIce/1 -> "EcuIce_facEtaCocMax_MAP "/2, Ice_tqLossesIce_MAP/2, Ice_relLoad2relTqOptIgnLamOne_MAP/2, Ice_relLoadMax_CUR/1, "EcuIce_facFuelEnRich_MAP "/2, EcuIce_tqLossesIce_MAP/2, EcuIce_facEtaCocMax_MAP/2, EcuIce_relTqOptIgnLamOne2Load_MAP/2, EcuIce_facFuelEnRich_MAP/2

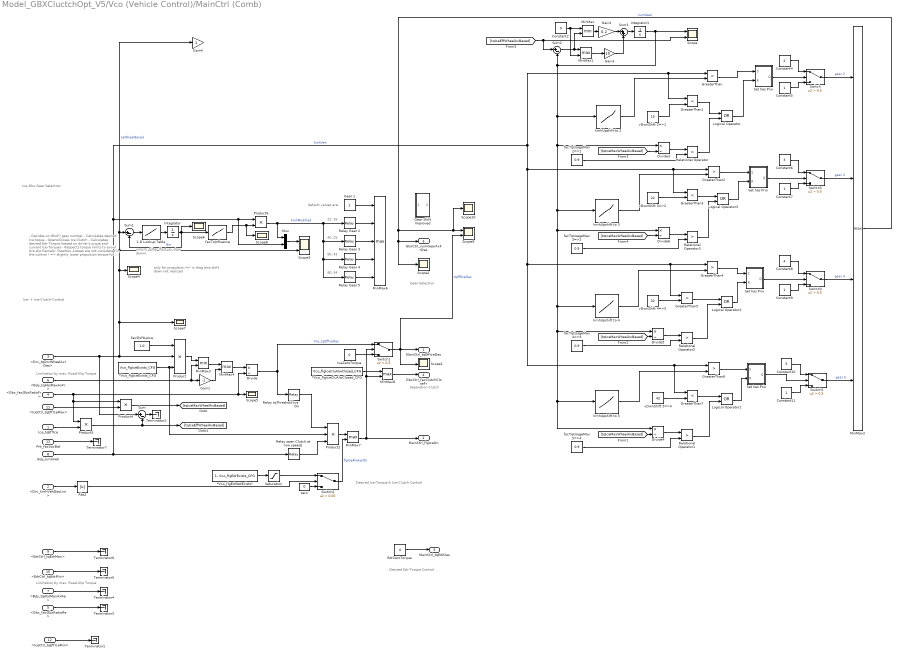
== system Model_GBXCluctchOpt_V5/Vco (Vehicle Control)/MainCtrl (Comb) ==
  note: default values are:
  note: unsym. Filter (fast up, slow down)
  note: only for propulsion
      | => in drag also shift down not realized
  note: 80..54
  note: 60..43
  note: 40..25
  note: 22..16
  note: Separation Clutch
  note: Gear Selection
  note: Limitation by max. Road-Slip Torque
  note: - Decides on GbxFr gear number
      | - Calculates desired Ice toque
      | - Opens/Closes Ice Clutch
      | - Calculates desired Edr-Torque
      |   (based on driver's orque and current Ice-Torque)
      | - Respects torque limits to avoid tire slip
      |
      | Remark:
      | Gearbox-Losses are not considered in the control !
      | => slightly lower propulsion torque for Edr and Ice
      | => also in torque limitation
  note: Desired Ice-Torque & Ice-Clutch Control
  note: Desired Edr-Torque Control
  note: Limitation by max. Road-Slip Torque
  note: Ice- + Ice-Clutch-Control
  note: Ice-Gbx Gear Selection
  Ice_tqEffIce : Inport
  <Drv_kmhVehDesLim> : Inport  Port=2
  <Drv_tqDrvWheelAxlDes> : Inport  Port=3
  <Gbx_facGbxRatioFr> : Inport  Port=4
  <Gbx_facGbxRatioRe> : Inport  Port=5
  <Bdy_tqAbsMaxAxFr> : Inport  Port=6
  <Bdy_tqAbsMaxAxRe> : Inport  Port=7
  Bdy_kmhVeh : Inport  Port=8
  <EdrCtrl_tqEdrMax> : Inport  Port=9
  <EdrCtrl_tqEdrMin> : Inport  Port=10
  <IceCtrl_tqEffIceMax> : Inport  Port=11
  <IceCtrl_tqEffIceMin> : Inport  Port=12
  Pnt_facSocBat : Inport  Port=13
  "  Set has Prio  " : Subsystem
  "*Vco_flgEdrNotExists\"" : Constant  Value=1- Vco_flgEdrExists_CFG
  *Vco_flgIceCluAlwClosed_CFG : Constant  Value=Vco_flgIceCluAlwClosed_CFG
  *Vco_flgIceExists_CFG : Constant  Value=Vco_flgIceExists_CFG
  1-D Lookup Table : Lookup_n-D  NumberOfTableDimensions=1  BreakpointsForDimension1="[-10000 0  10000]"  Table="[-2000   0 200000]"  InternalRulePriority=Speed  RndMeth=Simplest
  Abs2 : Abs  ZeroCross=off  SaturateOnIntegerOverflow=off
  Constant10 : Constant  Value=5
  Constant{5,7,9,11} (4 alike) : Constant
  Constant2 : Constant  Value=0
  Constant4 : Constant  Value=2
  Constant6 : Constant  Value=3
  Constant8 : Constant  Value=4
  Divide{,3..6} (5 alike) : Product  Inputs=*/
  EdrZeroTorque : Constant  Value=0
  Gain1 : Gain  Gain=-1
  Gain2 : Gain  Gain=0.2
  Gain3 : Gain  Gain=10
  Gain4 : Gain
  Gear 1 : Constant
  Gear Shift Improved : Subsystem
  GreaterThan{,2,4,6} (4 alike) : RelationalOperator  Operator=>  OutDataTypeStr=boolean  RndMeth=Simplest  InputSameDT=off
  GreaterThan{1,3,5,7} (4 alike) : RelationalOperator  Operator=<  OutDataTypeStr=boolean  RndMeth=Simplest  InputSameDT=off
  IceZeroTorque : Constant  Value=0
  Integrator : Integrator
  Integrator1 : Integrator
  Logical Operator{,1..3} (4 alike) : Logic  Operator=OR  AllPortsSameDT=off  OutDataTypeStr=boolean
  MinMax : MinMax  Inputs=2  ZeroCross=off
  MinMax{1,4,7..8} (4 alike) : MinMax  Function=max  Inputs=2  ZeroCross=off
  MinMax2 : MinMax  Function=max  Inputs=4
  MinMax3 : MinMax  Inputs=2
  MinMax6 : MinMax  Function=max  Inputs=5
  Mux : Mux  Inputs=2
  Product : Product  Inputs=3
  Product2 : Product  Inputs=3
  Product4 : Product
  Product5 : Product
  Product6 : Product
  Relational Operator{,1..3} (4 alike) : RelationalOperator  Operator=>  OutDataTypeStr=boolean  RndMeth=Simplest  InputSameDT=off
  Relay tqThreshold Ice On : Relay  OnSwitchValue=25  OffSwitchValue=17
  Relay Gear 2 : Relay  OnSwitchValue=22  OffSwitchValue=16  OnOutputValue=2
  Relay Gear 3 : Relay  OnSwitchValue=40  OffSwitchValue=25  OnOutputValue=3
  Relay Gear 4 : Relay  OnSwitchValue=60  OffSwitchValue=43  OnOutputValue=4
  Relay Gear 5 : Relay  OnSwitchValue=80  OffSwitchValue=54  OnOutputValue=5
  Relay open Clutch at low speeds : Relay  OnSwitchValue=11  OffSwitchValue=9
  Saturation : Saturate  UpperLimit=1  LowerLimit=0
  Scope : Scope  NumInputPorts=2
  Scope{1..2,4..8,10} (8 alike) : Scope
  Scope3 : Scope  NumInputPorts=2
  Scope9 : Scope  NumInputPorts=2
  Set has Prio : Subsystem
  "Set has Prio " : Subsystem
  "Set has Prio  " : Subsystem
  Sum : Sum  Inputs=|+-
  Sum1 : Sum  Inputs=|+-
  Sum2 : Sum  Inputs=|+-
  Sum3 : Sum  Inputs=|++
  Switch{,1,3..5} (5 alike) : Switch  Criteria=u2 > Threshold  Threshold=0.5  SaturateOnIntegerOverflow=off  InputSameDT=off
  Switch2 : Switch  Criteria=u2 > Threshold  Threshold=0.05  ZeroCross=off  SaturateOnIntegerOverflow=off  InputSameDT=off
  Terminator{1..7} (7 alike) : Terminator
  facShiftLpIce : Constant  Value=1.0
  facTqInfluence : Lookup_n-D  NumberOfTableDimensions=1  BreakpointsForDimension1="[0 10   500  1000   1500   2000   2500]"  Table="[1   1     0.9   0.8       0.7    0.6       0.5]"  ExtrapMethod=Clip  InternalRulePriority=Speed  RndMeth=Simplest
  facTqUsageMax 2=>1 : Constant  Value=0.9
  facTqUsageMax 3=>2 : Constant  Value=0.9
  facTqUsageMax 4=>3 : Constant  Value=0.9
  facTqUsageMax 5=>4 : Constant  Value=0.9
  kmhUpshift to 2 : Lookup_n-D  NumberOfTableDimensions=1  BreakpointsForDimension1="[0  1200  1700 5000]"  Table="[20  21      63  64]"  ExtrapMethod=Clip  InternalRulePriority=Speed  RndMeth=Simplest
  kmhUpshift to 3 : Lookup_n-D  NumberOfTableDimensions=1  BreakpointsForDimension1="[0  750  1250 5000]"  Table="[29  30      89  90]"  ExtrapMethod=Clip  InternalRulePriority=Speed  RndMeth=Simplest
  kmhUpshift to 4 : Lookup_n-D  NumberOfTableDimensions=1  BreakpointsForDimension1="[0  550  900 5000]"  Table="[40  41      126  127]"  ExtrapMethod=Clip  InternalRulePriority=Speed  RndMeth=Simplest
  kmhUpshift to 5 : Lookup_n-D  NumberOfTableDimensions=1  BreakpointsForDimension1="[0  420  650 5000]"  Table="[55  56      175  176]"  ExtrapMethod=Clip  InternalRulePriority=Speed  RndMeth=Simplest
  vDwnShift 2=>1 : Constant  Value=15
  vDwnShift 3=>2 : Constant  Value=22
  vDwnShift 4=>3 : Constant  Value=32
  vDwnShift 5=>4 : Constant  Value=42
  zero : Constant  Value=0
  MainCtrl_tqEffIceDes : Outport
  MainCtrl_flgIceOn : Outport  Port=2
  GbxCtrl_numGearAxFrDes : Outport  Port=3
  GbxCtrl_facClutchCloseFr : Outport  Port=4
  MainCtrl_tqEdrDes : Outport  Port=5
  wires:
  Divide/1 -> Relay tqThreshold Ice On/1, Switch1/1  "Vco_tqEffIceDes"
  <Gbx_facGbxRatioFr>/1 -> Scope5/1, Divide/2, Product4/1, Product5/1
  Product/1 -> MinMax3/1
  *Vco_flgIceExists_CFG/1 -> Product/3, Product2/2
  MinMax4/1 -> Divide/1
  <Bdy_tqAbsMaxAxFr>/1 -> MinMax3/2, Gain1/1
  MinMax3/1 -> MinMax4/1
  Gain1/1 -> MinMax4/2
  <IceCtrl_tqEffIceMax>/1 -> Product4/2
  <IceCtrl_tqEffIceMin>/1 -> Terminator1/1
  <Drv_kmhVehDesLim>/1 -> Abs2/1
  Abs2/1 -> Switch2/2
  Switch1/1 -> Scope9/2, Scope1/1, MainCtrl_tqEffIceDes/1  "tqEffIceDes"
  IceZeroTorque/1 -> Switch1/3
  Relay open Clutch at low speeds/1 -> Product2/3
  Sum/1 -> Terminator2/1
  Product5/1 -> [tqIceEffWheelAxBased], Sum/2
  Relay Gear 4/1 -> MinMax6/4
  Relay Gear 2/1 -> MinMax6/2
  Relay Gear 3/1 -> MinMax6/3
  Gear 1/1 -> MinMax6/1
  Product6/1 -> Relay Gear 2/1, Relay Gear 3/1, Relay Gear 4/1, Relay Gear 5/1, Mux/1  "kmhModified"
  facTqInfluence/1 -> Scope8/1, Product6/2
  Relay Gear 5/1 -> MinMax6/5
  Mux/1 -> Scope3/1
  Ice_tqEffIce/1 -> Product5/2
  MinMax7/1 -> Switch1/2, MinMax8/2, MainCtrl_flgIceOn/1
  Product2/1 -> MinMax7/1
  "*Vco_flgEdrNotExists\""/1 -> Saturation/1
  Switch2/1 -> MinMax7/2  "flgIceAlwaysOn"
  MinMax8/1 -> GbxCtrl_facClutchCloseFr/1
  *Vco_flgIceCluAlwClosed_CFG/1 -> MinMax8/1
  Saturation/1 -> Switch2/1
  zero/1 -> Switch2/3
  Sum1/1 -> 1-D Lookup Table/1
  1-D Lookup Table/1 -> Integrator/1
  Integrator/1 -> facTqInfluence/1, Scope6/1, Sum1/2  "Nm"
  facShiftLpIce/1 -> Product/1
  Relay tqThreshold Ice On/1 -> Product2/1
  EdrZeroTorque/1 -> MainCtrl_tqEdrDes/1
  <Gbx_facGbxRatioRe>/1 -> Terminator3/1
  <Bdy_tqAbsMaxAxRe>/1 -> Terminator4/1
  <EdrCtrl_tqEdrMin>/1 -> Terminator5/1
  <EdrCtrl_tqEdrMax>/1 -> Terminator6/1
  Pnt_facSocBat/1 -> Terminator7/1
  Set has Prio/1(Q) -> Switch/2
  Switch4/1 -> MinMax2/3  "gear 4"
  Switch3/1 -> MinMax2/2  "gear 3"
  MinMax2/1 -> Scope10/1, Scope9/1, GbxCtrl_numGearAxFrDes/1, Scope2/1  "numGear"
  GreaterThan6/1 -> "  Set has Prio  "/1(S)
  Constant9/1 -> Switch4/3
  Switch5/1 -> MinMax2/4  "gear 5"
  MinMax1/1 -> Gain3/1
  "Set has Prio  "/1(Q) -> Switch3/2
  "Set has Prio "/1(Q) -> Switch4/2
  Constant11/1 -> Switch5/3
  GreaterThan4/1 -> "Set has Prio "/1(S)
  Constant10/1 -> Switch5/1
  "  Set has Prio  "/1(Q) -> Switch5/2
  Constant6/1 -> Switch3/1
  GreaterThan2/1 -> "Set has Prio  "/1(S)
  Constant8/1 -> Switch4/1
  Constant7/1 -> Switch3/3
  Sum2/1 -> MinMax/2, MinMax1/1
  MinMax/1 -> Gain2/1
  Sum3/1 -> Integrator1/1
  Logical Operator/1 -> Set has Prio/2(R)
  Switch/1 -> MinMax2/1  "gear 2"
  Constant2/1 -> MinMax1/2, MinMax/1
  Constant5/1 -> Switch/3
  Gain2/1 -> Sum3/1
  Constant4/1 -> Switch/1
  GreaterThan/1 -> Set has Prio/1(S)
  <Drv_tqDrvWheelAxlDes>/1 -> Scope7/1, Scope4/1, Scope3/2, Gain4/1, Sum1/1, Product/2, Sum/1  "tqWheelBased"
  Gain3/1 -> Sum3/2
  kmhUpshift to 2/1 -> GreaterThan/2
  vDwnShift 2=>1/1 -> GreaterThan1/2
  kmhUpshift to 3/1 -> GreaterThan2/2
  kmhUpshift to 4/1 -> GreaterThan4/2
  kmhUpshift to 5/1 -> GreaterThan6/2
  Integrator1/1 -> Scope/1, kmhUpshift to 2/1, Divide3/1, kmhUpshift to 3/1, Divide6/1, kmhUpshift to 4/1, Divide5/1, kmhUpshift to 5/1, Divide4/1, Sum2/2
  vDwnShift 3=>2/1 -> GreaterThan3/2
  vDwnShift 4=>3/1 -> GreaterThan5/2
  vDwnShift 5=>4/1 -> GreaterThan7/2
  GreaterThan1/1 -> Logical Operator/1
  [tqIceMaxWheelAxBased] -> Divide3/2
  Divide3/1 -> Relational Operator/1
  facTqUsageMax 2=>1/1 -> Relational Operator/2
  Relational Operator/1 -> Logical Operator/2
  facTqUsageMax 5=>4/1 -> Relational Operator1/2
  [tqIceMaxWheelAxBased] -> Divide4/2
  Divide4/1 -> Relational Operator1/1
  Relational Operator1/1 -> Logical Operator1/2
  GreaterThan7/1 -> Logical Operator1/1
  Logical Operator1/1 -> "  Set has Prio  "/2(R)
  Logical Operator2/1 -> "Set has Prio "/2(R)
  GreaterThan5/1 -> Logical Operator2/1
  Relational Operator2/1 -> Logical Operator2/2
  Divide5/1 -> Relational Operator2/1
  facTqUsageMax 4=>3/1 -> Relational Operator2/2
  [tqIceMaxWheelAxBased] -> Divide5/2
  Product4/1 -> [tqIceMaxWheelAxBased]
  GreaterThan3/1 -> Logical Operator3/1
  Logical Operator3/1 -> "Set has Prio  "/2(R)
  Relational Operator3/1 -> Logical Operator3/2
  Divide6/1 -> Relational Operator3/1
  [tqIceMaxWheelAxBased] -> Divide6/2
  facTqUsageMax 3=>2/1 -> Relational Operator3/2
  Bdy_kmhVeh/1 -> GreaterThan3/1, GreaterThan2/1, GreaterThan5/1, GreaterThan4/1, GreaterThan6/1, GreaterThan7/1, GreaterThan1/1, GreaterThan/1, Product6/1, Mux/2, Relay open Clutch at low speeds/1  "kmhVeh"
  [tqIceEffWheelAxBased] -> Sum2/1, Scope/2
